simulink model "frbd_64ch_600mhz"  (R2013b)
(part 4 of 149)

  Constant100/1 -> ACC9/3(we)
  edge_detect9/1 -> Counter17/1, Accumulator9/2
  adder_tree9/1(sync_out) -> Accumulator9/3, edge_detect9/1
  adder_tree9/2(dout) -> Accumulator9/1
  Register9/1 -> [frb_detector_10]
  [cnt_rst] -> Register9/2
  Relational29/1 -> Register9/3, Register9/1
  Accumulator9/1 -> Relational29/2, ACC10/2(data_in)
  Counter17/1 -> ACC10/1(addr)
  ACC10/1(data_out) -> Terminator40/1
  pipeline255/1(q) -> adder_tree9/2(din1)
  pipeline256/1(q) -> adder_tree9/3(din2)
  pipeline257/1(q) -> adder_tree9/4(din3)
  pipeline258/1(q) -> adder_tree9/5(din4)
  theta10/1(in_reg) -> Convert10/1
  Convert10/1 -> Relational29/1
  pipeline252/1(q) -> adder_tree9/1(sync)
  Constant102/1 -> ACC10/3(we)
  pipeline37/1(q) -> adder_tree10/2(din1)
  pipeline42/1(q) -> adder_tree10/3(din2)
  pipeline53/1(q) -> adder_tree10/4(din3)
  pipeline55/1(q) -> adder_tree10/5(din4)
  Constant104/1 -> ACC0/3(we)
  pipeline93/1(q) -> pipeline40/1(d), pipeline44/1(d), pipeline27/1(d), pipeline30/1(d), pipeline39/1(d)
  pipeline98/1(q) -> pipeline22/1(d), pipeline19/1(d), pipeline17/1(d), pipeline15/1(d), pipeline20/1(d)
  pipeline111/1(q) -> pipeline13/1(d)
  pipeline113/1(q) -> pipeline14/1(d)
  pipeline143/1(q) -> pipeline16/1(d)
  pipeline145/1(q) -> pipeline18/1(d)
  pipeline179/1(q) -> pipeline12/1(d)
  pipeline184/1(q) -> pipeline25/1(d)
  pipeline195/1(q) -> pipeline28/1(d)
  pipeline197/1(q) -> pipeline38/1(d)
  pipeline240/1(q) -> pipeline68/1(d)
  pipeline291/1(q) -> pipeline74/1(d), pipeline73/1(d), pipeline71/1(d), pipeline69/1(d), pipeline76/1(d)
  pipeline251/1(q) -> pipeline70/1(d)
  pipeline253/1(q) -> pipeline72/1(d)
  pipeline235/1(q) -> pipeline66/1(d)
  pipeline325/1(q) -> pipeline79/1(d)
  pipeline353/1(q) -> pipeline100/1(d), pipeline81/1(d), pipeline95/1(d), pipeline84/1(d), pipeline96/1(d)
  pipeline327/1(q) -> pipeline82/1(d)
  pipeline296/1(q) -> pipeline65/1(d)
  pipeline352/1(q) -> pipeline94/1(d)
  pipeline355/1(q) -> pipeline158/1(d)
  pipeline357/1(q) -> pipeline162/1(d)
  pipeline356/1(q) -> pipeline160/1(d)
  pipeline354/1(q) -> pipeline157/1(d)
  pipeline358/1(q) -> pipeline164/1(d), pipeline161/1(d), pipeline163/1(d), pipeline159/1(d), pipeline166/1(d)
  pipeline359/1(q) -> pipeline152/1(d)
  pipeline361/1(q) -> pipeline172/1(d)
  pipeline360/1(q) -> pipeline169/1(d)
  pipeline362/1(q) -> pipeline180/1(d)
  pipeline363/1(q) -> pipeline186/1(d), pipeline171/1(d), pipeline181/1(d), pipeline174/1(d), pipeline182/1(d)
  pipeline368/1(q) -> pipeline218/1(d), pipeline211/1(d), pipeline215/1(d), pipeline213/1(d), pipeline216/1(d)
  pipeline365/1(q) -> pipeline210/1(d)
  pipeline364/1(q) -> pipeline208/1(d)
  pipeline367/1(q) -> pipeline214/1(d)
  pipeline366/1(q) -> pipeline212/1(d)
  pipeline372/1(q) -> pipeline236/1(d)
  pipeline370/1(q) -> pipeline221/1(d)
  pipeline373/1(q) -> pipeline238/1(d), pipeline237/1(d), pipeline226/1(d), pipeline223/1(d), pipeline125/1(d)
  pipeline371/1(q) -> pipeline224/1(d)
  pipeline369/1(q) -> pipeline207/1(d)
  pipeline376/1(q) -> pipeline272/1(d)
  pipeline375/1(q) -> pipeline270/1(d)
  pipeline377/1(q) -> pipeline274/1(d)
  pipeline378/1(q) -> pipeline276/1(d), pipeline275/1(d), pipeline273/1(d), pipeline271/1(d), pipeline278/1(d)
  pipeline374/1(q) -> pipeline269/1(d)
  pipeline382/1(q) -> pipeline292/1(d)
  pipeline381/1(q) -> pipeline284/1(d)
  pipeline379/1(q) -> pipeline268/1(d)
  pipeline380/1(q) -> pipeline281/1(d)
  pipeline383/1(q) -> pipeline293/1(d), pipeline286/1(d), pipeline283/1(d), pipeline242/1(d), pipeline294/1(d)
  pipeline387/1(q) -> pipeline340/1(d)
  pipeline386/1(q) -> pipeline338/1(d)
  pipeline388/1(q) -> pipeline342/1(d), pipeline341/1(d), pipeline339/1(d), pipeline337/1(d), pipeline316/1(d)
  pipeline384/1(q) -> pipeline335/1(d)
  pipeline385/1(q) -> pipeline336/1(d)
  pipeline389/1(q) -> pipeline617/1(d)
  pipeline391/1(q) -> pipeline606/1(d)
  pipeline392/1(q) -> pipeline604/1(d)
  pipeline390/1(q) -> pipeline601/1(d)
  pipeline393/1(q) -> pipeline605/1(d), pipeline607/1(d), pipeline603/1(d), pipeline625/1(d), pipeline624/1(d)
  pipeline397/1(q) -> pipeline306/1(d)
  pipeline394/1(q) -> pipeline311/1(d)
  pipeline396/1(q) -> pipeline308/1(d)
  pipeline395/1(q) -> pipeline303/1(d)
  pipeline398/1(q) -> pipeline314/1(d), pipeline307/1(d), pipeline309/1(d), pipeline305/1(d), pipeline315/1(d)
  [m0d0] -> Delay13/1
  [m0d1] -> Delay8/1
  [m0d2] -> Delay21/1
  [m0d3] -> Delay30/1
  [m0d4] -> Delay39/1
  [m0d5] -> Delay56/1
  [m0d6] -> Delay44/1
  [m0d7] -> Delay51/1
  [m0d8] -> Delay59/1
  [m0d9] -> Delay66/1
  [m0d10] -> Delay81/1
  [m0d11] -> Delay119/1
  Mult/1 -> m0_tree/1(In1)
  pipeline350/1(q) -> sync_tree/1(In1)
  Mult1/1 -> m1_tree/1(In1)
  Mult2/1 -> m2_tree/1(In1)
  Mult3/1 -> m3_tree/1(In1)
  [sd0] -> Delay12/1
  [m1d0] -> Delay33/1
  [m2d0] -> Delay35/1
  [m3d0] -> Delay37/1
  [sd1] -> Delay5/1
  [m1d1] -> Delay10/1
  [m2d1] -> Delay14/1
  [m3d1] -> Delay15/1
  [sd2] -> Delay19/1
  [m1d2] -> Delay26/1
  [m2d2] -> Delay27/1
  [m3d2] -> Delay28/1
  [sd3] -> Delay29/1
  [m1d3] -> Delay18/1
  [m2d3] -> Delay24/1
  [m3d3] -> Delay25/1
  [sd4] -> Delay32/1
  [m1d4] -> Delay52/1
  [m2d4] -> Delay53/1
  [m3d4] -> Delay54/1
  [sd5] -> Delay55/1
  [m1d5] -> Delay31/1
  [m2d5] -> Delay40/1
  [m3d5] -> Delay41/1
  [sd6] -> Delay43/1
  [m1d6] -> Delay47/1
  [m2d6] -> Delay48/1
  [m3d6] -> Delay49/1
  [sd7] -> Delay50/1
  [m1d7] -> Delay42/1
  [m2d7] -> Delay45/1
  [m3d7] -> Delay46/1
  [sd8] -> Delay58/1
  [m1d8] -> Delay62/1
  [m2d8] -> Delay63/1
  [m3d8] -> Delay64/1
  [sd9] -> Delay65/1
  [m1d9] -> Delay57/1
  [m2d9] -> Delay60/1
  [m3d9] -> Delay61/1
  [sd10] -> Delay80/1
  [m1d10] -> Delay77/1
  [m2d10] -> Delay78/1
  [m3d10] -> Delay79/1
  [sd11] -> Delay127/1
  [m1d11] -> Delay120/1
  [m2d11] -> Delay121/1
  [m3d11] -> Delay122/1
  [rst] -> pipeline421/1
  [rst] -> pipeline422/1
  [gbe_data] -> pipeline423/1
  [gbe_valid] -> pipeline424/1
  [gbe_eof] -> pipeline430/1
  Constant105/1 -> one_GbE/8
  [gbe_dest_ip] -> pipeline428/1
  [gbe_dest_port] -> pipeline429/1
  one_GbE/1 -> Terminator59/1
  one_GbE/2 -> Terminator60/1
  one_GbE/3 -> Terminator61/1
  one_GbE/4 -> Terminator53/1
  one_GbE/5 -> Terminator54/1
  one_GbE/6 -> Terminator55/1
  one_GbE/7 -> Terminator56/1
  one_GbE/8 -> Terminator57/1
  one_GbE/9 -> Terminator58/1
  one_GbE/10 -> Terminator51/1
  one_GbE/11 -> Terminator52/1
  Concat/1 -> pipeline406/1
  ring/1(dout) -> pipeline403/1
  ring/2(eof) -> pipeline404/1
  ring/3(val) -> pipeline405/1
  pipeline407/1 -> Concat/1
  pipeline408/1 -> Concat/2
  pipeline409/1 -> Concat/3
  pipeline406/1 -> ring/2(data_in)
  [adc0_a] -> pipeline407/1
  [adc0_c] -> pipeline408/1
  [adc1_a] -> pipeline409/1
  gbe_dest_port/1(in_reg) -> Delay92/1
  gbe_dest_ip/1(in_reg) -> Delay91/1
  control/1(in_reg) -> Slice3/1, Slice2/1, Slice1/1
  Slice1/1 -> Delay86/1
  Slice2/1 -> Delay87/1
  Delay86/1 -> [write]
  Delay87/1 -> [rst]
  pipeline298/1 -> [adc1_a], [adc0_c], [adc0_a]
  conv_bus0/9(q8) -> pipeline298/1
  pipeline299/1 -> pipeline8/1(d), bus_create0/8(in8)
  pipeline300/1 -> pipeline7/1(d), bus_create0/7(in7)
  pipeline301/1 -> pipeline1/1(d), bus_create0/1(in1)
  pipeline349/1 -> pipeline2/1(d), bus_create0/2(in2)
  pipeline399/1 -> pipeline3/1(d), bus_create0/3(in3)
  pipeline400/1 -> pipeline4/1(d), bus_create0/4(in4)
  pipeline401/1 -> pipeline5/1(d), bus_create0/5(in5)
  pipeline402/1 -> pipeline6/1(d), bus_create0/6(in6)
  Slice3/1 -> Delay88/1
  [frb_detector_0] -> pipeline420/1
  [frb_detector_1] -> pipeline419/1
  [frb_detector_2] -> pipeline418/1
  [frb_detector_3] -> pipeline417/1
  [frb_detector_4] -> pipeline416/1
  [frb_detector_5] -> pipeline415/1
  [frb_detector_6] -> pipeline414/1
  [frb_detector_7] -> pipeline413/1
  [frb_detector_8] -> pipeline412/1
  [frb_detector_9] -> pipeline411/1
  [frb_detector_10] -> pipeline410/1
  Concat1/1 -> Convert/1
  Convert/1 -> frb_detector/1(out_reg)
  Logical/1 -> pipeline/1
  Delay88/1 -> [allow_detect]
  [detection] -> Delay93/1
  [write] -> Logical24/2
  Logical23/1 -> Logical24/1
  [allow_detect] -> Inverter/1
  Logical24/1 -> gpio1/1, ring/1(write_en)
  Inverter/1 -> Logical23/1
  pipeline403/1 -> [gbe_data]
  pipeline404/1 -> [gbe_eof]
  pipeline405/1 -> [gbe_valid]
  Delay91/1 -> [gbe_dest_ip]
  Delay92/1 -> [gbe_dest_port]
  Delay93/1 -> Logical23/2
  pipeline/1 -> gpio/1, [detection]
  pipeline410/1 -> Logical/1, Concat1/1
  pipeline411/1 -> Logical/2, Concat1/2
  pipeline412/1 -> Logical/3, Concat1/3
  pipeline413/1 -> Logical/4, Concat1/4
  pipeline414/1 -> Logical/5, Concat1/5
  pipeline415/1 -> Logical/6, Concat1/6
  pipeline416/1 -> Logical/7, Concat1/7
  pipeline417/1 -> Logical/8, Concat1/8
  pipeline418/1 -> Logical/9, Concat1/9
  pipeline419/1 -> Logical/10, Concat1/10
  pipeline420/1 -> Logical/11, Concat1/11
  pipeline421/1 -> one_GbE/1
  pipeline422/1 -> one_GbE/2
  pipeline423/1 -> one_GbE/3
  pipeline424/1 -> one_GbE/4
  pipeline428/1 -> one_GbE/5
  pipeline429/1 -> one_GbE/6
  pipeline430/1 -> one_GbE/7
  Logical1/1 -> Parallel_Dedispersor_v11/2(Data1)
  BitBasher/1 -> Logical1/1
  BitBasher1/1 -> Logical3/1
  BitBasher2/1 -> Logical5/1
  Logical5/1 -> Parallel_Dedispersor_v11/4(Data3)
  BitBasher3/1 -> Logical7/1
  Logical7/1 -> Parallel_Dedispersor_v11/5(Data4)
  BitBasher4/1 -> Logical9/1
  BitBasher5/1 -> Logical11/1
  BitBasher6/1 -> Logical13/1
  BitBasher7/1 -> Logical15/1
  BitBasher8/1 -> Logical17/1
  BitBasher9/1 -> Logical19/1
  BitBasher10/1 -> Logical21/1
  BitBasher11/1 -> Logical25/1
  BitBasher12/1 -> Logical26/1
  BitBasher13/1 -> Logical27/1
  BitBasher14/1 -> Logical28/1
  BitBasher15/1 -> Logical29/1
  BitBasher16/1 -> Logical30/1
  BitBasher17/1 -> Logical31/1
  BitBasher18/1 -> Logical32/1
  BitBasher19/1 -> Logical33/1
  BitBasher20/1 -> Logical34/1
  BitBasher21/1 -> Logical35/1
  BitBasher22/1 -> Logical36/1
  Logical37/1 -> Parallel_Dedispersor_v5/5(Data4)
  BitBasher23/1 -> Logical37/1
  BitBasher24/1 -> Logical38/1
  BitBasher25/1 -> Logical39/1
  Logical40/1 -> Parallel_Dedispersor_v6/4(Data3)
  BitBasher26/1 -> Logical40/1
  Logical41/1 -> Parallel_Dedispersor_v6/5(Data4)
  BitBasher27/1 -> Logical41/1
  BitBasher28/1 -> Logical42/1
  Logical42/1 -> Parallel_Dedispersor_v7/2(Data1)
  Logical43/1 -> Parallel_Dedispersor_v7/3(Data2)
  BitBasher29/1 -> Logical43/1
  Logical44/1 -> Parallel_Dedispersor_v7/4(Data3)
  BitBasher30/1 -> Logical44/1
  Logical45/1 -> Parallel_Dedispersor_v7/5(Data4)
  BitBasher31/1 -> Logical45/1
  BitBasher32/1 -> Logical46/1
  Logical46/1 -> Parallel_Dedispersor_v8/2(Data1)
  Logical47/1 -> Parallel_Dedispersor_v8/3(Data2)
  BitBasher33/1 -> Logical47/1
  Logical48/1 -> Parallel_Dedispersor_v8/4(Data3)
  BitBasher34/1 -> Logical48/1
  Logical49/1 -> Parallel_Dedispersor_v8/5(Data4)
  BitBasher35/1 -> Logical49/1
  BitBasher36/1 -> Logical50/1
  Logical50/1 -> Parallel_Dedispersor_v9/2(Data1)
  Logical51/1 -> Parallel_Dedispersor_v9/3(Data2)
  BitBasher37/1 -> Logical51/1
  Logical52/1 -> Parallel_Dedispersor_v9/4(Data3)
  BitBasher38/1 -> Logical52/1
  Logical53/1 -> Parallel_Dedispersor_v9/5(Data4)
  BitBasher39/1 -> Logical53/1
  BitBasher40/1 -> Logical54/1
  BitBasher41/1 -> Logical55/1
  Logical56/1 -> pipeline331/1(d)
  BitBasher42/1 -> Logical56/1
  Logical57/1 -> pipeline332/1(d)
  BitBasher43/1 -> Logical57/1
